simulink model "TESAOffense50Day2"  (R2025b)
settings: Solver=FixedStepAuto  StartTime=0.0  StopTime=SimulationTime  FixedStep=timestep  RelTol=1e-3
model workspace (MAT data in the model file):
  alt_init = Simulink.Parameter
  alt_init.Value = 0
  alt_init.Complexity = 'real'
  alt_init.Dimensions = [1 1]
  alt_init.DataType = 'auto'
  fense_lats = Simulink.Parameter
  fense_lats.Value = [14.2944040379 14.3012064984]
  fense_lats.Complexity = 'real'
  fense_lats.Dimensions = [1 2]
  fense_lats.DataType = 'auto'
  fense_lons = Simulink.Parameter
  fense_lons.Value = [101.167230479 101.176793822]
  fense_lons.Complexity = 'real'
  fense_lons.Dimensions = [1 2]
  fense_lons.DataType = 'auto'
  lat_init = Simulink.Parameter
  lat_init.Value = 14.30312811
  lat_init.Complexity = 'real'
  lat_init.Dimensions = [1 1]
  lat_init.DataType = 'auto'
  long_init = Simulink.Parameter
  long_init.Value = 101.154574732
  long_init.Complexity = 'real'
  long_init.Dimensions = [1 1]
  long_init.DataType = 'auto'
values from neighbouring files (symbols this model uses):
  g = [0;0;g0]    [Quadrotor_Drone_PD_Control.m]
  m = 0.468    [Quadrotor_Drone_PD_Control.m]
undefined symbols (not defined in the file or in its folder): dspblkCoreblockFVToolHelper, fractalcoef, gcbh, I, K
libraries: dspstat3 x5, dspfdesign x1, sensorgpslib x1, mspsensorlib x1, matrix_library x1
settings Model: Creator=worap  LastModifiedBy=Sitasen
settings DataIOCC: ExternalInput=inputStructure  LoadExternalInput=on
settings ConfigSetCC: MQTTTableInfo=[]

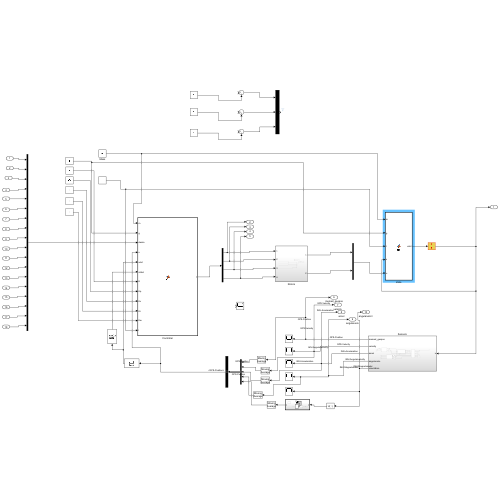
[thumbnail: Simulink's stored preview of the top-level diagram]
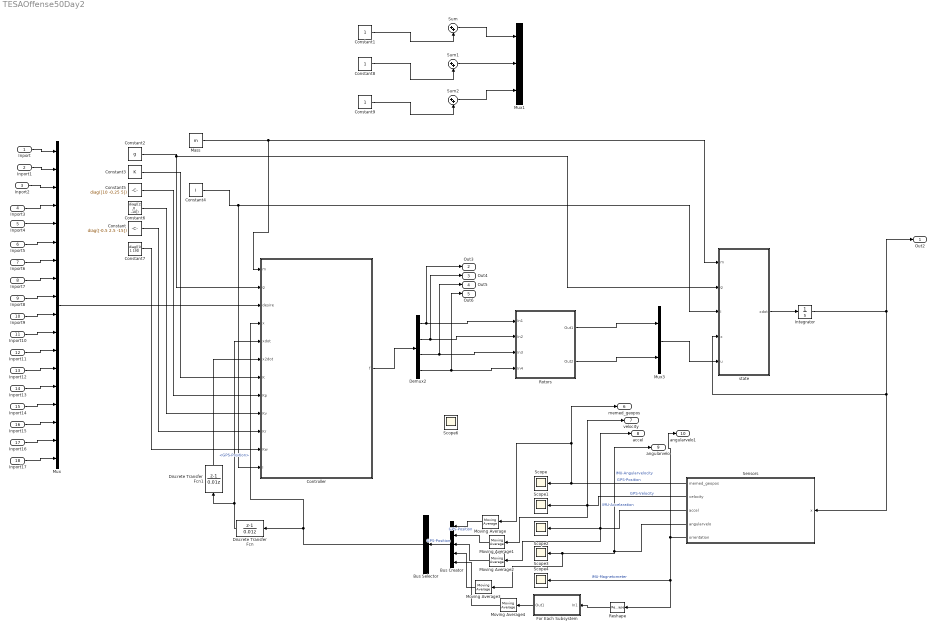
== system TESAOffense50Day2 ==
  Inport : Inport
  Inport1 : Inport  Port=2
  Inport2 : Inport  Port=3
  Inport3 : Inport  Port=4
  Inport4 : Inport  Port=5
  Inport5 : Inport  Port=6
  Inport6 : Inport  Port=7
  Inport7 : Inport  Port=8
  Inport8 : Inport  Port=9
  Inport9 : Inport  Port=10
  Inport10 : Inport  Port=11
  Inport11 : Inport  Port=12
  Inport12 : Inport  Port=13
  Inport13 : Inport  Port=14
  Inport14 : Inport  Port=15
  Inport15 : Inport  Port=16
  Inport16 : Inport  Port=17
  Inport17 : Inport  Port=18
  Bus Creator : BusCreator  Inputs=5
  Bus Selector : BusSelector  OutputSignals=GPS-Position
  Constant : Constant  Value=diag([-0.5 2.5 -15])
  Constant1 : Constant
  Constant2 : Constant  Value=g
  Constant3 : Constant  Value=K
  Constant4 : Constant  Value=I
  Constant5 : Constant  Value=diag([10 -0.25 5])
  Constant6 : Constant  Value=diag([2 ,0 , -10])
  Constant7 : Constant  Value=diag([0 1 19])
  Constant8 : Constant
  Constant9 : Constant
  Controller : MATLAB Function  TreatAsAtomicUnit=on
  Demux2 : Demux
  Discrete Transfer Fcn : DiscreteTransferFcn  LoadFcn=dspblkCoreblockFVToolHelper(gcbh,'load');  Numerator=[1 -1]  Denominator=[0.01 0]
      settings: CopyFcn=dspblkCoreblockFVToolHelper(gcbh,'copy');  DeleteFcn=dspblkCoreblockFVToolHelper(gcbh,'close');  ModelCloseFcn=dspblkCoreblockFVToolHelper(gcbh,'close');  PreSaveFcn=dspblkCoreblockFVToolHelper(gcbh,'presave');  PostSaveFcn=dspblkCoreblockFVToolHelper(gcbh,'postsave');  CloseFcn=dspblkCoreblockFVToolHelper(gcbh,'close');
  Discrete Transfer Fcn1 : DiscreteTransferFcn  LoadFcn=dspblkCoreblockFVToolHelper(gcbh,'load');  Numerator=[1 -1]  Denominator=[0.01 0]
      settings: CopyFcn=dspblkCoreblockFVToolHelper(gcbh,'copy');  DeleteFcn=dspblkCoreblockFVToolHelper(gcbh,'close');  ModelCloseFcn=dspblkCoreblockFVToolHelper(gcbh,'close');  PreSaveFcn=dspblkCoreblockFVToolHelper(gcbh,'presave');  PostSaveFcn=dspblkCoreblockFVToolHelper(gcbh,'postsave');  CloseFcn=dspblkCoreblockFVToolHelper(gcbh,'close');
  For Each Subsystem : Subsystem  TreatAsAtomicUnit=on
  Integrator : Integrator  InitialCondition=[0;0;0;0;0;0;1;0;0;0;1;0;0;0;1;0;0;0]
  Mass : Constant  Value=m
  Moving Average{,1..4} (5 alike) : dspstat3/Moving Average  Method=Sliding window  ForgettingFactorPort=off  SpecifyWindowLength=on  WindowLength=4  OverlapLength=3  AllowArbitraryInputLength=off  ForgettingFactor=0.9  SimulateUsing=Interpreted execution
  Mux : Mux  Inputs=18
  Mux1 : Mux  Inputs=3
  Mux3 : Mux  Inputs=2
  Reshape : Reshape
  Rotors : Subsystem
  Scope{,1..4,6} (6 alike) : Scope
      Scope settings: ActiveDisplayYMinimum=-137.09622866734583  ActiveDisplayYMaximum=94.399855381105411
      Scope1 settings: ActiveDisplayYMinimum=-279.21758887442786  ActiveDisplayYMaximum=485.12005268873543  DataLoggingVariableName=ScopeData2
      Scope2 settings: ActiveDisplayYMinimum=-439.87620375239328  ActiveDisplayYMaximum=411.06315254108921  DataLoggingVariableName=ScopeData3
      Scope3 settings: ActiveDisplayYMinimum=-1.1945655208409198  ActiveDisplayYMaximum=1.01043447915908  DataLoggingVariableName=ScopeData4
      Scope4 settings: ActiveDisplayYMinimum=-0.78481865815606378  ActiveDisplayYMaximum=0.94285653890688814  DataLoggingVariableName=ScopeData5
      Scope6 settings: ActiveDisplayYMinimum=-0.10349  ActiveDisplayYMaximum=2.21622
  Sensors : Subsystem
  Sum : Sum  Inputs=|++
  Sum1 : Sum  Inputs=|++
  Sum2 : Sum  Inputs=|++
  state : MATLAB Function  TreatAsAtomicUnit=on
  Out2 : Outport
  Out3 : Outport  Port=2
  Out4 : Outport  Port=3
  Out5 : Outport  Port=4
  Out6 : Outport  Port=5
  memed_geopos : Outport  Port=6
  velocity : Outport  Port=7
  accel : Outport  Port=8
  angularvelo : Outport  Port=9
  angularvelo1 : Outport  Port=10
  wires:
  Mass/1 -> state/1(m), Controller/1(m)
  Demux2/2 -> Out4/1, Rotors/2(In2)
  Rotors/1(Out1) -> Mux3/1
  Rotors/2(Out2) -> Mux3/2
  Demux2/3 -> Out5/1, Rotors/3(In3)
  Demux2/4 -> Out6/1, Rotors/4(In4)
  Constant4/1 -> state/3(I), Controller/12(I)
  Controller/1(f) -> Demux2/1
  Demux2/1 -> Out3/1, Rotors/1(In1)
  Constant2/1 -> state/2(g), Controller/2(g)
  Constant3/1 -> Controller/7(K)
  Constant5/1 -> Controller/8(Kp)
  Constant6/1 -> Controller/9(Kv)
  Constant7/1 -> Controller/11(Kw)
  Constant/1 -> Controller/10(Kr)
  Mux3/1 -> state/5(u)
  state/1(xdot) -> Integrator/1
  Mux/1 -> Controller/3(desire)
  Inport17/1 -> Mux/18
  Inport16/1 -> Mux/17
  Inport15/1 -> Mux/16
  Inport14/1 -> Mux/15
  Inport13/1 -> Mux/14
  Inport12/1 -> Mux/13
  Inport11/1 -> Mux/12
  Inport10/1 -> Mux/11
  Inport9/1 -> Mux/10
  Inport8/1 -> Mux/9
  Inport7/1 -> Mux/8
  Inport6/1 -> Mux/7
  Inport5/1 -> Mux/6
  Inport4/1 -> Mux/5
  Inport3/1 -> Mux/4
  Inport1/1 -> Mux/2
  Inport2/1 -> Mux/3
  Discrete Transfer Fcn1/1 -> Controller/6(x2dot)
  Bus Creator/1 -> Bus Selector/1  "GPS-Position"
  Sensors/5(orientation) -> Scope4/1, Reshape/1, angularvelo1/1  "IMU-Magnetometer"
  Sensors/4(angularvelo) -> Scope3/1, Moving Average3/1, angularvelo/1  "IMU-Angularvelocity"
  Sensors/3(accel) -> accel/1, Moving Average2/1, Scope2/1  "IMU-Accelaration"
  Sensors/2(velocity) -> velocity/1, Moving Average1/1, Scope1/1  "GPS-Velocity"
  Sensors/1(memed_geopos) -> Moving Average/1, memed_geopos/1, Scope/1  "GPS-Position"
  Integrator/1 -> Sensors/1(x), state/4(x), Out2/1
  Discrete Transfer Fcn/1 -> Controller/5(xdot), Discrete Transfer Fcn1/1
  Bus Selector/1 -> Controller/4(x), Discrete Transfer Fcn/1  "<GPS-Position>"
  Moving Average/1 -> Bus Creator/1  "GPS-Position"
  Moving Average1/1 -> Bus Creator/2
  Moving Average2/1 -> Bus Creator/3
  Moving Average3/1 -> Bus Creator/4
  Moving Average4/1 -> Bus Creator/5
  Reshape/1 -> For Each Subsystem/1(In1)
  For Each Subsystem/1(Out1) -> Moving Average4/1
  Sum2/1 -> Mux1/3
  Sum1/1 -> Mux1/2
  Constant9/1 -> Sum2/2
  Constant1/1 -> Sum/2
  Sum/1 -> Mux1/1
  Constant8/1 -> Sum1/2
  Inport/1 -> Mux/1

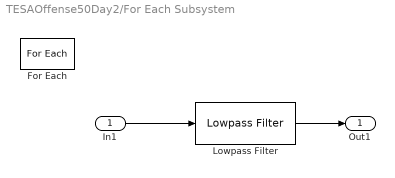
== system TESAOffense50Day2/For Each Subsystem ==
  In1 : Inport  Partition=on  PartitionDimension=1  PartitionWidth=1  PartitionOffset=0
  For Each : ForEach  DisableCoverage=on
  Lowpass Filter : dspfdesign/Lowpass Filter  FilterType=FIR  DesignForMinimumOrder=on  FilterOrder=50  PassbandFrequency=0.3628  StopbandFrequency=0.5442  PassbandRipple=0.1  StopbandAttenuation=80  SampleRateMode=Use normalized frequency (0 to 1)  SampleRate=44100  SimulateUsing=Interpreted execution  roundingMode=Floor  coeffsDataTypeStr=fixdt(1,16)
  Out1 : Outport  ConcatenationDimension=1
  wires:
  In1/1 -> Lowpass Filter/1
  Lowpass Filter/1 -> Out1/1

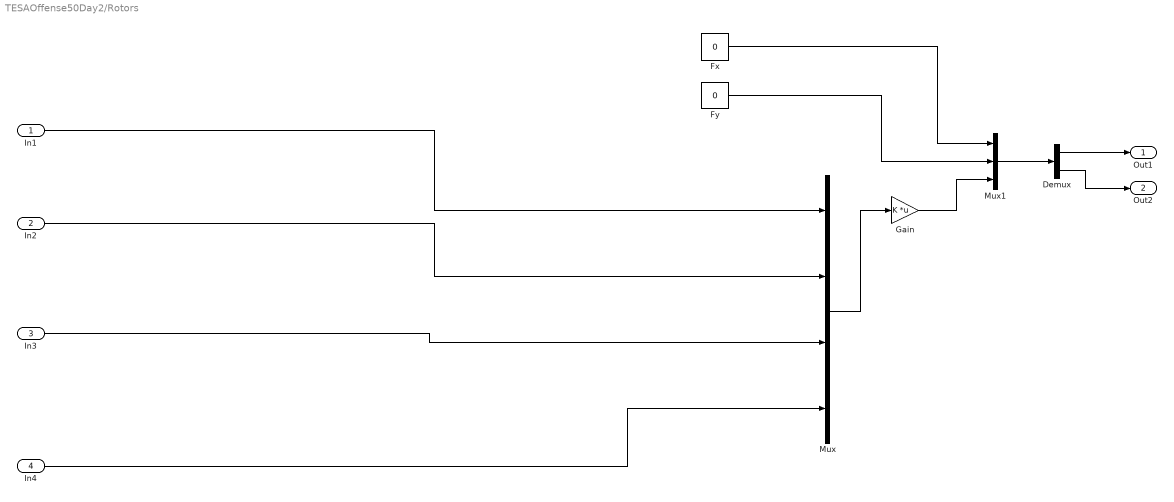
== system TESAOffense50Day2/Rotors ==
  In1 : Inport
  In2 : Inport  Port=2
  In3 : Inport  Port=3
  In4 : Inport  Port=4
  Demux : Demux  Outputs=2
  Fx : Constant  Value=0
  Fy : Constant  Value=0
  Gain : Gain  Gain=K  Multiplication=Matrix(K*u) (u vector)
  Mux : Mux
  Mux1 : Mux  Inputs=3
  Out1 : Outport
  Out2 : Outport  Port=2
  wires:
  Fx/1 -> Mux1/1
  Mux1/1 -> Demux/1
  Fy/1 -> Mux1/2
  Mux/1 -> Gain/1
  Gain/1 -> Mux1/3
  Demux/2 -> Out2/1
  Demux/1 -> Out1/1
  In1/1 -> Mux/1
  In2/1 -> Mux/2
  In3/1 -> Mux/3
  In4/1 -> Mux/4

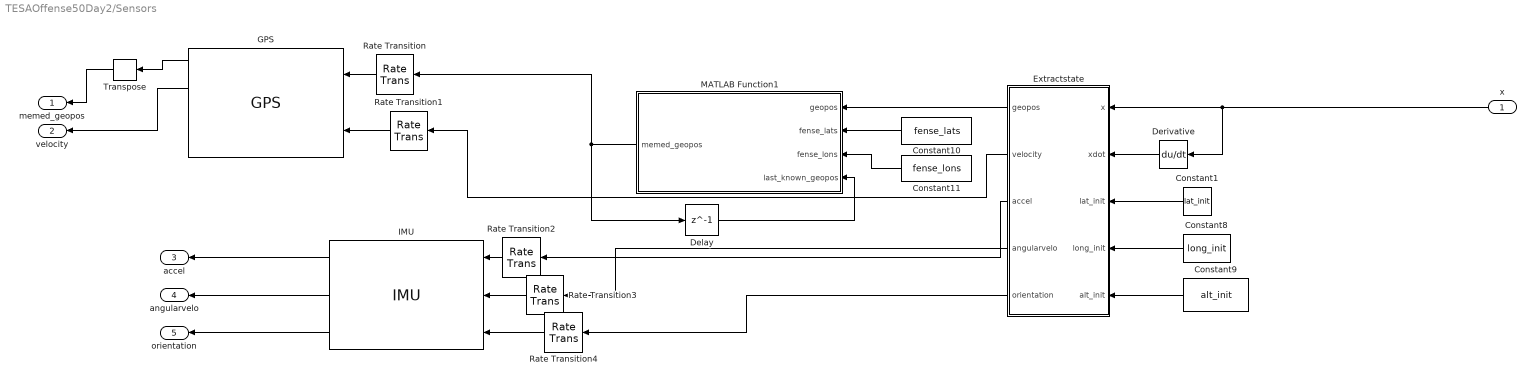
== system TESAOffense50Day2/Sensors ==
  x : Inport
  Constant1 : Constant  Value=lat_init
  Constant10 : Constant  Value=fense_lats
  Constant11 : Constant  Value=fense_lons
  Constant8 : Constant  Value=long_init
  Constant9 : Constant  Value=alt_init
  Delay : Delay  DelayLength=1  InitialCondition=0
  Derivative : Derivative
  Extractstate : MATLAB Function  TreatAsAtomicUnit=on
  GPS : sensorgpslib/GPS  DispRefFrame=NED  PositionInputFormat=Geodetic  ReferenceLocation=[ 0, 0, 0 ]  HorizontalPositionAccuracy=1.6  VerticalPositionAccuracy=3  VelocityAccuracy=0.1  DecayFactor=0.999  SeedDouble=67  SimulateUsing=Interpreted execution
      settings: LibrarySourceBlock=mspsensorlib/GPS
  IMU : mspsensorlib/IMU  DispRefFrame=NED  TemperaturePort=off  Temperature=25  MagneticFieldPort=off  MagneticFieldNED=[ 27.5550, -2.4169, -16.0849 ]  MagneticFieldENU=[ -2.4169, 27.5550, 16.0849 ]  SeedDouble=67  SimulateUsing=Interpreted execution  AccelParamsMeasurementRange=Inf  AccelParamsResolution=0  AccelParamsConstantBias=[ 0, 0, 0 ]  AccelParamsAxesMisalignment=[ 100, 0, 0; 0, 100, 0; 0, 0, 100 ]  AccelParamsNoiseDensity=[ 0.003924 0.003924 0.003924 ]  AccelParamsBiasInstability=[ 0, 0, 0 ]  AccelParamsBiasInstabilityNumerator=fractalcoef().Numerator  AccelParamsBiasInstabilityDenominator=fractalcoef().Denominator  AccelParamsRandomWalk=[ 0, 0, 0 ]  AccelParamsNoiseType=double-sided  AccelParamsTemperatureBias=[ 0, 0, 0 ]  AccelParamsTemperatureScaleFactor=[ 0, 0, 0 ]  GyroParamsMeasurementRange=Inf  GyroParamsResolution=0  GyroParamsConstantBias=[ 0, 0, 0 ]  GyroParamsAxesMisalignment=[ 100, 0, 0; 0, 100, 0; 0, 0, 100 ]  GyroParamsAccelerationBias=[ 0, 0, 0 ]  GyroParamsNoiseDensity=[ 0.0125, 0.0125, 0.0125 ]  GyroParamsBiasInstability=[ 0, 0, 0 ]  GyroParamsBiasInstabilityNumerator=fractalcoef().Numerator  GyroParamsBiasInstabilityDenominator=fractalcoef().Denominator  GyroParamsRandomWalk=[ 0, 0, 0 ]  GyroParamsNoiseType=double-sided  GyroParamsTemperatureBias=[ 0, 0, 0 ]  GyroParamsTemperatureScaleFactor=[ 0, 0, 0 ]  MagParamsMeasurementRange=Inf  MagParamsResolution=0  MagParamsConstantBias=[ 0, 0, 0 ]  MagParamsAxesMisalignment=[ 100, 0, 0; 0, 100, 0; 0, 0, 100 ]  MagParamsNoiseDensity=[0.6 0.6 0.9]/sqrt(100)  MagParamsBiasInstability=[ 0, 0, 0 ]  MagParamsBiasInstabilityNumerator=fractalcoef().Numerator  MagParamsBiasInstabilityDenominator=fractalcoef().Denominator  MagParamsRandomWalk=[ 0, 0, 0 ]  MagParamsNoiseType=double-sided  MagParamsTemperatureBias=[ 0, 0, 0 ]  MagParamsTemperatureScaleFactor=[ 0, 0, 0 ]
  MATLAB Function1 : MATLAB Function  TreatAsAtomicUnit=on
  Rate Transition{,1..4} (5 alike) : RateTransition
  Transpose : matrix_library/Transpose
  memed_geopos : Outport
  velocity : Outport  Port=2
  accel : Outport  Port=3
  angularvelo : Outport  Port=4
  orientation : Outport  Port=5
  wires:
  Constant11/1 -> MATLAB Function1/3(fense_lons)
  Constant8/1 -> Extractstate/4(long_init)
  Constant1/1 -> Extractstate/3(lat_init)
  Constant10/1 -> MATLAB Function1/2(fense_lats)
  Delay/1 -> MATLAB Function1/4(last_known_geopos)
  Derivative/1 -> Extractstate/2(xdot)
  Constant9/1 -> Extractstate/5(alt_init)
  Extractstate/1(geopos) -> MATLAB Function1/1(geopos)
  MATLAB Function1/1(memed_geopos) -> Delay/1, Rate Transition/1
  x/1 -> Derivative/1, Extractstate/1(x)
  IMU/1 -> accel/1
  IMU/2 -> angularvelo/1
  IMU/3 -> orientation/1
  Extractstate/3(accel) -> Rate Transition2/1
  Extractstate/4(angularvelo) -> Rate Transition3/1
  Extractstate/5(orientation) -> Rate Transition4/1
  Extractstate/2(velocity) -> Rate Transition1/1
  GPS/1 -> Transpose/1
  GPS/2 -> velocity/1
  Rate Transition/1 -> GPS/1
  Rate Transition1/1 -> GPS/2
  Rate Transition2/1 -> IMU/1
  Rate Transition3/1 -> IMU/2
  Rate Transition4/1 -> IMU/3
  Transpose/1 -> memed_geopos/1

== matlab function TESAOffense50Day2/state ==
  data: m input; g input; I input; x input; u input; xdot output
function xdot = fcn(m,g,I,x,u)

% extract the x-vextor
p = x(1:3,1);
v = x(4:6,1);
R = reshape(x(7:15,1),3,3);
omega = x(16:18,1);

%control signal
f = u(3,1);
M = u(4:6,1);

e3 = [0;0;1];


xdot = zeros(size(x));

xdot(1:3,1) = v;
xdot(4:6,1) = g*e3 - 1/m*f*R*e3;

Rdot = R*hatmap(omega);
xdot(7:15,1) = Rdot(:);

xdot(16:18,1) = I\(M - cross(omega,I*omega));




end

== matlab function TESAOffense50Day2/Controller ==
  data: m input; g input; f output; desire input; x input; xdot input; x2dot input; K input; Kp input; Kv input; Kr input; Kw input; I input
function f   = fcn(m,g,desire,x,xdot,x2dot,K,Kp,Kv,Kr,Kw,I)

% persistent r2dot_prev;
% if isempty(r2dot_prev)
%     r2dot_prev = [0;0;0];
% end
tolerance = 1e-6;

vee_map = @(M) [M(3,2); M(1,3); M(2,1)];

xt = desire(1);
yt = desire(2) ;
zt = desire(3);

dxt = desire(4);
dyt = desire(5);
dzt = desire(6);

ddxt = desire(7);
ddyt = desire(8);
ddzt = desire(9);

dddxt = desire(10);
dddyt = desire(11);
dddzt = desire(12); 
ddddxt = desire(13);
ddddyt = desire(14);
ddddzt = desire(15);

psit = desire(16);
dpsit = desire(17);
ddpsit = desire(18);
r_current = x(1:3);
v_current = [dxt;dyt;dzt];
R = reshape([ddxt; ddyt; ddzt; dddxt; dddyt; dddzt; ddddxt; ddddyt; ddddzt], 3, 3);
%d_R xdot
%dd_R x2dot
omega = [psit; dpsit; ddpsit];
rd = [xt;yt;zt];
dv = [dxt;dyt;dzt];
da = [ddxt;ddyt;ddzt];
e3 = [0; 0; 1];
trajectory = [xt;yt;zt;psit];

%{
att = x(4:6);    % [phi; theta; psi]
phi = att(1);
theta = att(2);
psi = att(3);

c_phi = cos(phi); s_phi = sin(phi);
c_th = cos(theta); s_th = sin(theta);
c_psi = cos(psi); s_psi = sin(psi);

% --- 3. คำนวณเมทริกซ์การหมุนปัจจุบัน (R) ---
R = [c_psi*c_th, c_psi*s_th*s_phi - s_psi*c_phi, c_psi*s_th*c_phi + s_psi*s_phi;
     s_psi*c_th, s_psi*s_th*s_phi + c_psi*c_phi, s_psi*s_th*c_phi - c_psi*s_phi;
     -s_th,      c_th*s_phi,                    c_th*c_phi];

%}
%%ส่วน2
ex = r_current - rd;
ev = v_current - dv;

%ส่วน1
dd_xd = x2dot(1);

F_des_vec = - (-Kp * ex - Kv * ev + m * g * e3 + dd_xd);
F_des_norm = norm(F_des_vec);




if F_des_norm < tolerance
    z_Bdes = e3;
else
    z_Bdes = F_des_vec / F_des_norm;
end


h = [cos(psit); sin(psit); 0];
y_Bdes_unnormalized = cross(z_Bdes, h);
y_Bdes_norm = norm(y_Bdes_unnormalized);
if y_Bdes_norm < tolerance
    % avoid singularity
    temp_vec = cross(e3, z_Bdes);
    if norm(temp_vec) < tolerance
        y_Bdes = [0;1;0];
    else
        y_Bdes = temp_vec / norm(temp_vec);
    end
else
    y_Bdes = y_Bdes_unnormalized / y_Bdes_norm;
end

x_Bdes = cross(y_Bdes, z_Bdes);

Rd = [x_Bdes, y_Bdes, z_Bdes];

 

f_total = F_des_vec' *R *e3;
% if f_total < 0
%     f_total = 0;
% end

eR_matrix = 0.5 * (Rd' * R - R' * Rd);
eR = vee_map(eR_matrix);

omega_d_des_body_frame = [0; 0; dpsit];
e_omega = omega - R' * Rd * omega_d_des_body_frame; 

M = -Kr * eR - Kw * e_omega + cross(omega, I * omega);
u = [f_total; M];
f = K \ u;

% f(f < 0) = 0;

display(f_total);

end

== matlab function TESAOffense50Day2/Sensors/Extractstate ==
  data: geopos output; velocity output; x input; accel output; xdot input; angularvelo output; orientation output; lat_init input; long_init input; alt_init input
function [geopos, velocity,accel, angularvelo, orientation] = Extractstate(x,xdot,lat_init,long_init,alt_init)

position = x(1:3)';
velocity = x(4:6)';
accel = xdot(4:6)';
R = x(7:15);
orientation = reshape(R,3,3);
angularvelo = x(16:18)';


geopos = ned2lla(position, [lat_init long_init alt_init], "ellipsoid");

end

== matlab function TESAOffense50Day2/Sensors/MATLAB Function1 ==
  data: geopos input; memed_geopos output; fense_lats input; fense_lons input; last_known_geopos input
function memed_geopos  = is_jammed(geopos, fense_lats, fense_lons, last_known_geopos)
    
    memed_geopos = geopos;

    if fense_lats ~= 0
        if (geopos(1) > min(fense_lats)) && (geopos(1) < max(fense_lats)) && (geopos(2) > min(fense_lons)) && (geopos(2) < max(fense_lons))
            memed_geopos = [14.30613815134626, 101.18904132968885, 30];
        end
    end
end
